simulink model "HH_curremt"  (R2020b)
settings: Solver=VariableStepAuto  StartTime=0.0  StopTime=10.0  RelTol=1e-3
values from neighbouring files (symbols this model uses):
  capa = 1    [solver.m]
  G_K_max = 36    [solver.m]
  G_L = 0.3    [HH_model.m]    (also in HH_model_proto.m; scratch.m; solver.m)
  G_Na_max = 120    [solver.m]
  h0 = 1    [solver.m]
  m0 = 0    [solver.m]
  n0 = 0    [solver.m]
  V_K = -12    [solver.m]
  V_L = 10.613    [solver.m]
  V_Na = 115    [solver.m]
settings Model: Creator=haedongkim  LastModifiedBy=haedo
settings SFSimCC: CustomCodeUndefinedFunction=UseInterfaceOnly

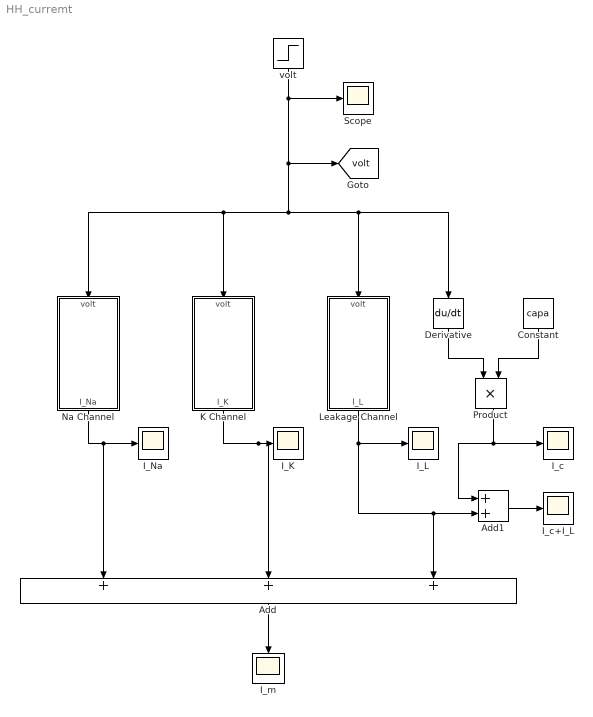
== system HH_curremt ==
  Add : Sum  Inputs=+++
  Add1 : Sum
  Constant : Constant  Value=capa
  Derivative : Derivative
  I_K : Scope
  I_L : Scope
  I_Na : Scope
  I_c : Scope
  I_c+I_L : Scope
  I_m : Scope
  K Channel : Subsystem
  Leakage Channel : Subsystem
  Na Channel : Subsystem
  Product : Product
  Scope : Scope
  volt : Step  Before=-65  After=20  SampleTime=0.001
  tag scope: volt=global
  wires:
  Na Channel/1(I_Na) -> I_Na/1, Add/1
  K Channel/1(I_K) -> I_K/1, Add/2
  Leakage Channel/1(I_L) -> I_L/1, Add1/2, Add/3
  Derivative/1 -> Product/1
  Constant/1 -> Product/2
  Product/1 -> Add1/1, I_c/1
  volt/1 -> [volt], Leakage Channel/1(volt), Derivative/1, K Channel/1(volt), Na Channel/1(volt), Scope/1
  Add/1 -> I_m/1
  Add1/1 -> I_c+I_L/1

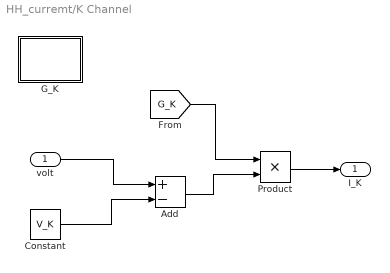
== system HH_curremt/K Channel ==
  volt : Inport
  Add : Sum  Inputs=+-
  Constant : Constant  Value=V_K
  G_K : Subsystem
  Product : Product
  I_K : Outport  VectorParamsAs1DForOutWhenUnconnected=off
  wires:
  volt/1 -> Add/1
  Constant/1 -> Add/2
  [G_K] -> Product/1
  Add/1 -> Product/2
  Product/1 -> I_K/1

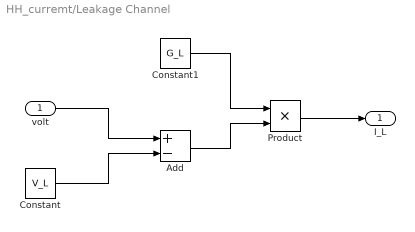
== system HH_curremt/Leakage Channel ==
  volt : Inport
  Add : Sum  Inputs=+-
  Constant : Constant  Value=V_L
  Constant1 : Constant  Value=G_L
  Product : Product
  I_L : Outport  VectorParamsAs1DForOutWhenUnconnected=off
  wires:
  volt/1 -> Add/1
  Constant/1 -> Add/2
  Add/1 -> Product/2
  Constant1/1 -> Product/1
  Product/1 -> I_L/1

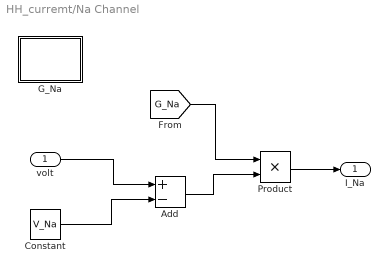
== system HH_curremt/Na Channel ==
  volt : Inport
  Add : Sum  Inputs=+-
  Constant : Constant  Value=V_Na
  G_Na : Subsystem
  Product : Product
  I_Na : Outport  VectorParamsAs1DForOutWhenUnconnected=off
  wires:
  volt/1 -> Add/1
  Constant/1 -> Add/2
  [G_Na] -> Product/1
  Add/1 -> Product/2
  Product/1 -> I_Na/1

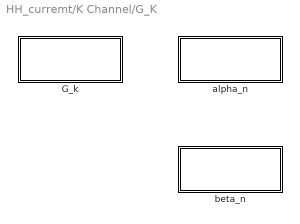
== system HH_curremt/K Channel/G_K ==
  G_k : Subsystem
  alpha_n : Subsystem
  beta_n : Subsystem

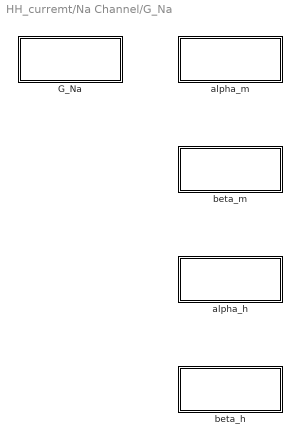
== system HH_curremt/Na Channel/G_Na ==
  G_Na : Subsystem
  alpha_h : Subsystem
  alpha_m : Subsystem
  beta_h : Subsystem
  beta_m : Subsystem

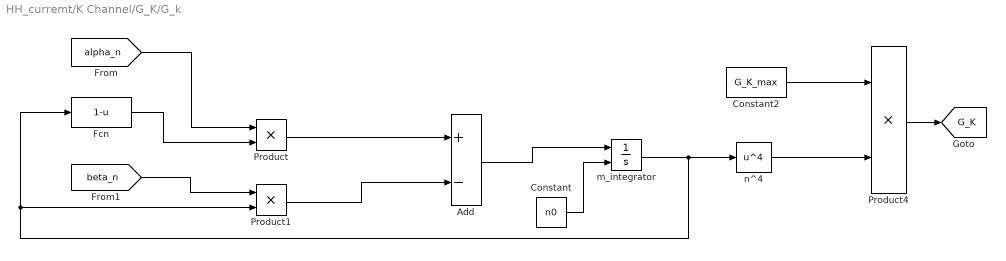
== system HH_curremt/K Channel/G_K/G_k ==
  Add : Sum  Inputs=+-
  Constant : Constant  Value=n0
  Constant2 : Constant  Value=G_K_max
  Fcn : Fcn  Expr=1-u
  Product : Product
  Product1 : Product
  Product4 : Product
  m_integrator : Integrator  InitialConditionSource=external
  n^4 : Fcn  Expr=u^4
  tag scope: G_K=global
  wires:
  [alpha_n] -> Product/1
  [beta_n] -> Product1/1
  Product/1 -> Add/1
  Product1/1 -> Add/2
  Add/1 -> m_integrator/1
  Constant/1 -> m_integrator/2
  m_integrator/1 -> n^4/1, Fcn/1, Product1/2
  n^4/1 -> Product4/2
  Constant2/1 -> Product4/1
  Product4/1 -> [G_K]
  Fcn/1 -> Product/2

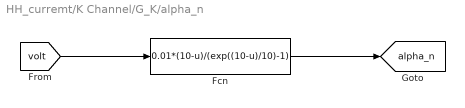
== system HH_curremt/K Channel/G_K/alpha_n ==
  Fcn : Fcn  Expr=0.01*(10-u)/(exp((10-u)/10)-1)
  tag scope: alpha_n=global
  wires:
  Fcn/1 -> [alpha_n]
  [volt] -> Fcn/1

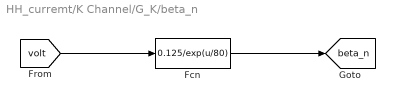
== system HH_curremt/K Channel/G_K/beta_n ==
  Fcn : Fcn  Expr=0.125/exp(u/80)
  tag scope: beta_n=global
  wires:
  [volt] -> Fcn/1
  Fcn/1 -> [beta_n]

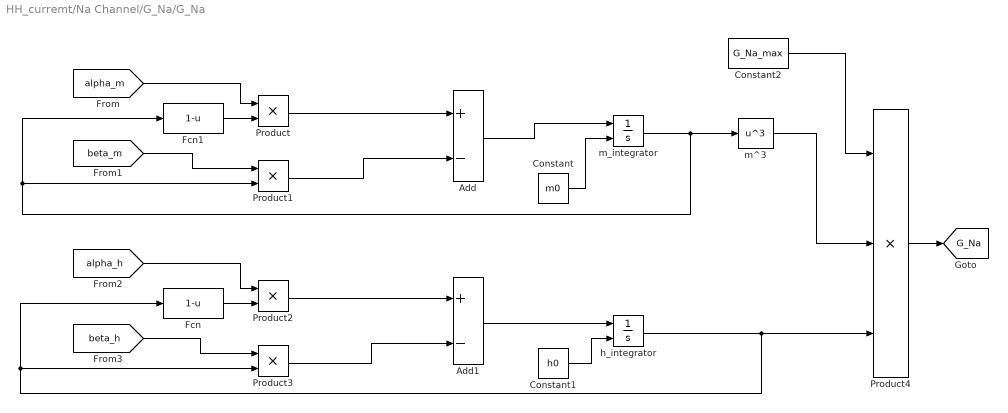
== system HH_curremt/Na Channel/G_Na/G_Na ==
  Add : Sum  Inputs=+-
  Add1 : Sum  Inputs=+-
  Constant : Constant  Value=m0
  Constant1 : Constant  Value=h0
  Constant2 : Constant  Value=G_Na_max
  Fcn : Fcn  Expr=1-u
  Fcn1 : Fcn  Expr=1-u
  Product{,1..3} (4 alike) : Product
  Product4 : Product  Inputs=3
  h_integrator : Integrator  InitialConditionSource=external
  m^3 : Fcn  Expr=u^3
  m_integrator : Integrator  InitialConditionSource=external
  tag scope: G_Na=global
  wires:
  [alpha_m] -> Product/1
  [beta_m] -> Product1/1
  Product/1 -> Add/1
  Product1/1 -> Add/2
  [alpha_h] -> Product2/1
  [beta_h] -> Product3/1
  Product3/1 -> Add1/2
  Product2/1 -> Add1/1
  Add/1 -> m_integrator/1
  Constant/1 -> m_integrator/2
  m_integrator/1 -> m^3/1, Fcn1/1, Product1/2
  Add1/1 -> h_integrator/1
  Constant1/1 -> h_integrator/2
  m^3/1 -> Product4/2
  h_integrator/1 -> Product3/2, Fcn/1, Product4/3
  Constant2/1 -> Product4/1
  Product4/1 -> [G_Na]
  Fcn1/1 -> Product/2
  Fcn/1 -> Product2/2

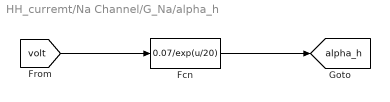
== system HH_curremt/Na Channel/G_Na/alpha_h ==
  Fcn : Fcn  Expr=0.07/exp(u/20)
  tag scope: alpha_h=global
  wires:
  [volt] -> Fcn/1
  Fcn/1 -> [alpha_h]

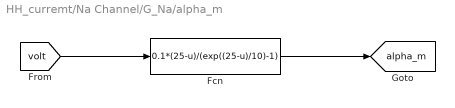
== system HH_curremt/Na Channel/G_Na/alpha_m ==
  Fcn : Fcn  Expr=0.1*(25-u)/(exp((25-u)/10)-1)
  tag scope: alpha_m=global
  wires:
  Fcn/1 -> [alpha_m]
  [volt] -> Fcn/1

== system HH_curremt/Na Channel/G_Na/beta_h ==
  Fcn : Fcn  Expr=1/(exp((30-u)/10)+1)
  tag scope: beta_h=global
  wires:
  [volt] -> Fcn/1
  Fcn/1 -> [beta_h]

== system HH_curremt/Na Channel/G_Na/beta_m ==
  Fcn : Fcn  Expr=4/exp(u/18)
  tag scope: beta_m=global
  wires:
  [volt] -> Fcn/1
  Fcn/1 -> [beta_m]
